simulink model "testRollContSolo"  (R2014a)
settings: Solver=ode3  StartTime=0.0  StopTime=20  FixedStep=0.021  RelTol=1e-3
values from neighbouring files (symbols this model uses):
  armLength = 0.23    [RollDynamics.m]    (also in RollDynamicsPWM-Theta.m; rollDynamics.m)
  enableSaturation = -1    [RollDynamics.m]
  Kforce = Ct*rho*Aprop*2*Whovering*Radius^2    (= 0.344086923283)    [RollDynamics.m]    (also in rollDynamics.m)
  mode = 1    [RollDynamics.m]    (also in RollDynamicsPWM-Theta.m = -1; rollDynamics.m = -1)
  pwmLowerBound = 1001    [RollDynamics.m]    (also in RollDynamicsPWM-Theta.m = 1100; rollDynamics.m = 1000)
  pwmUpperBound = 2000    [RollDynamics.m]    (also in RollDynamicsPWM-Theta.m = 1700; rollDynamics.m = 1800)
  Ts = 0.021    [RollDynamics.m]    (also in RollDynamicsPWM-Theta.m; rollDynamics.m)
  Whovering = 1420    [RollDynamics.m]    (also in RollDynamicsPWM-Theta.m = 750; rollDynamics.m)
undefined symbols (not defined in the file or in its folder): motor_den_tf_discrete, motor_num_tf_discrete, roll_den_tf_discrete, sigbuilder_block
libraries: simulink x2
settings Model: Creator=root  LastModifiedBy=root

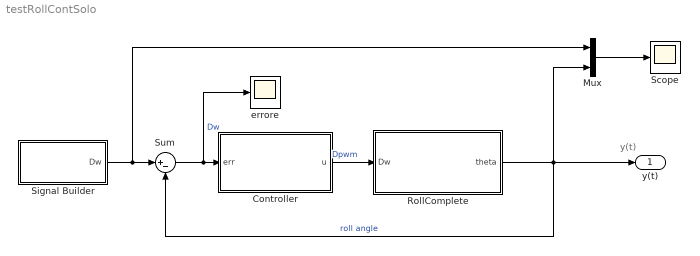
== system testRollContSolo ==
  note: y(t)
  "Controller " : Subsystem
  Mux : Mux  Inputs=2
  "RollComplete " : Subsystem
  Scope : Scope
      settings: TimeRange=10  YMin=-4  YMax=11
  Signal Builder : Subsystem  Tag=STV Subsys  LoadFcn=sigbuilder_block('load');  StartFcn=sigbuilder_block('start');  StopFcn=sigbuilder_block('stop');  ClipboardFcn=sigbuilder_block('clipboard');  mask(Sigbuilder block){}
      mask help: Simulink:masks:SigbuilderBlock_MD
      mask init:
      | if ~strcmp(get_param(bdroot(gcbh),'SimulationStatus'),'stopped') tuvar = sigbuilder_block('maskInit'); end
      settings: CopyFcn=sigbuilder_block('copy');  DeleteFcn=sigbuilder_block('delete');  ModelCloseFcn=sigbuilder_block('modelClose');  PreSaveFcn=sigbuilder_block('preSave');  PauseFcn=sigbuilder_block('pause');  ContinueFcn=sigbuilder_block('continue');  NameChangeFcn=sigbuilder_block('namechange');  OpenFcn=sigbuilder_block('open',[264.8 0 542.4 376 ]);  CloseFcn=sigbuilder_block('close');
      mask Display: plot(0, 0, 100, 100,[2, 2, 32, 32, 2], [68, 8, 8, 68, 68],[32, 2], [38, 38], [32, 19, 2],[53, 60, 44], [32, 17, 17, 2],[16, 16, 31, 31]);txt = getActiveGroup(gcbh);text(2, 100, txt,'verticalAlignment', 'top');
  Sum : Sum  Inputs=|+-
  errore : Scope
      settings: TimeRange=10  YMin=-4  YMax=11
  y(t) : Outport
  wires:
  Signal Builder/1(Dw) -> Mux/1, Sum/1
  Mux/1 -> Scope/1
  "RollComplete "/1("theta ") -> Sum/2, Mux/2, y(t)/1  "roll angle"
  Sum/1 -> errore/1, "Controller "/1("err ")  "Dw"
  "Controller "/1("u ") -> "RollComplete "/1("Dw ")  "Dpwm"

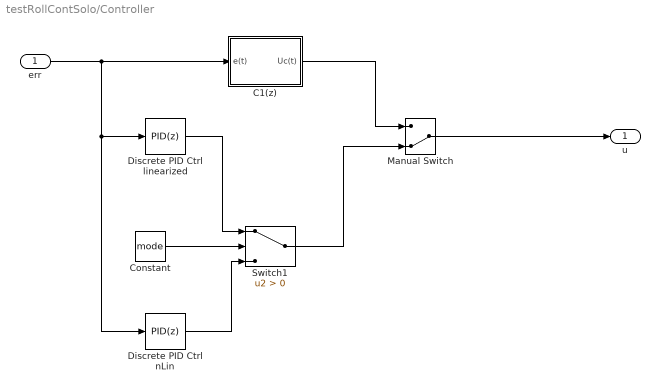
== system testRollContSolo/Controller  ==
  "err " : Inport
  C1(z) : Subsystem
  Constant : Constant  Value=mode
  Discrete PID Ctrl nLin : simulink/Continuous/PID Controller  Controller=PID  TimeDomain=Discrete-time  SampleTime=Ts  IntegratorMethod=Forward Euler  FilterMethod=Forward Euler  Form=Parallel  P=10000  I=0  D=0  N=16.4030945436849  InitialConditionSource=internal  InitialConditionForIntegrator=0  InitialConditionForFilter=0  ExternalReset=none  LimitOutput=off  UpperSaturationLimit=inf  LowerSaturationLimit=-inf  LinearizeAsGain=off  AntiWindupMode=none  Kb=1  TrackingMode=off  Kt=1  PParamMin=[]  PParamMax=[]  IParamMin=[]  IParamMax=[]  DParamMin=[]  DParamMax=[]  NParamMin=[]  NParamMax=[]  KbParamMin=[]  KbParamMax=[]  KtParamMin=[]  KtParamMax=[]  POutMin=[]  POutMax=[]  IOutMin=[]  IOutMax=[]  DOutMin=[]  DOutMax=[]  NOutMin=[]  NOutMax=[]  KbOutMin=[]  KbOutMax=[]  KtOutMin=[]  KtOutMax=[]  IntegratorOutMin=[]  IntegratorOutMax=[]  FilterOutMin=[]  FilterOutMax=[]  SumOutMin=[]  SumOutMax=[]  SumI1OutMin=[]  SumI1OutMax=[]  SumI2OutMin=[]  SumI2OutMax=[]  SumI3OutMin=[]  SumI3OutMax=[]  SumDOutMin=[]  SumDOutMax=[]  SaturationOutMin=[]  SaturationOutMax=[]  IntegratorContinuousStateAttributes=''  IntegratorStateMustResolveToSignalObject=off  IntegratorRTWStateStorageClass=Auto  FilterContinuousStateAttributes=''  FilterStateMustResolveToSignalObject=off  FilterRTWStateStorageClass=Auto
  "Discrete PID Ctrl linearized " : simulink/Continuous/PID Controller  Controller=PID  TimeDomain=Discrete-time  SampleTime=Ts  IntegratorMethod=Forward Euler  FilterMethod=Forward Euler  Form=Parallel  P=54.1819263876867  I=60.1281255168025  D=11.2520369375895  N=27.8352283138862  InitialConditionSource=internal  InitialConditionForIntegrator=0  InitialConditionForFilter=0  ExternalReset=none  LimitOutput=on  UpperSaturationLimit=pwmUpperBound  LowerSaturationLimit=pwmLowerBound  LinearizeAsGain=off  AntiWindupMode=back-calculation  Kb=1  TrackingMode=off  Kt=1  PParamMin=[]  PParamMax=[]  IParamMin=[]  IParamMax=[]  DParamMin=[]  DParamMax=[]  NParamMin=[]  NParamMax=[]  KbParamMin=[]  KbParamMax=[]  KtParamMin=[]  KtParamMax=[]  POutMin=[]  POutMax=[]  IOutMin=[]  IOutMax=[]  DOutMin=[]  DOutMax=[]  NOutMin=[]  NOutMax=[]  KbOutMin=[]  KbOutMax=[]  KtOutMin=[]  KtOutMax=[]  IntegratorOutMin=[]  IntegratorOutMax=[]  FilterOutMin=[]  FilterOutMax=[]  SumOutMin=[]  SumOutMax=[]  SumI1OutMin=[]  SumI1OutMax=[]  SumI2OutMin=[]  SumI2OutMax=[]  SumI3OutMin=[]  SumI3OutMax=[]  SumDOutMin=[]  SumDOutMax=[]  SaturationOutMin=[]  SaturationOutMax=[]  IntegratorContinuousStateAttributes=''  IntegratorStateMustResolveToSignalObject=off  IntegratorRTWStateStorageClass=Auto  FilterContinuousStateAttributes=''  FilterStateMustResolveToSignalObject=off  FilterRTWStateStorageClass=Auto
  Manual Switch : ManualSwitch  CurrentSetting=0
  Switch1 : Switch  Criteria=u2 > Threshold
  "u " : Outport
  wires:
  "err "/1 -> Discrete PID Ctrl nLin/1, "Discrete PID Ctrl linearized "/1, C1(z)/1(e(t))
  Manual Switch/1 -> "u "/1
  Discrete PID Ctrl nLin/1 -> Switch1/3
  C1(z)/1(Uc(t)) -> Manual Switch/1
  "Discrete PID Ctrl linearized "/1 -> Switch1/1
  Constant/1 -> Switch1/2
  Switch1/1 -> Manual Switch/2

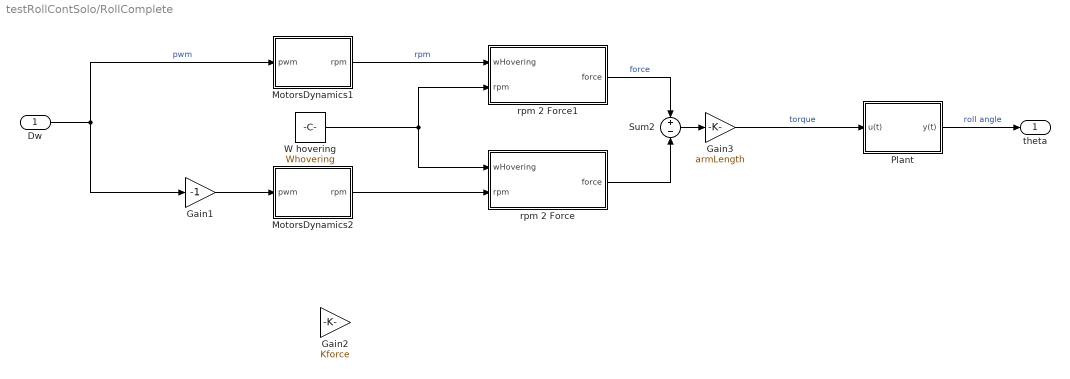
== system testRollContSolo/RollComplete  ==
  "Dw " : Inport
  Gain1 : Gain  Gain=-1  SampleTime=Ts
  Gain2 : Gain  Gain=Kforce  SampleTime=Ts
  Gain3 : Gain  Gain=armLength  SampleTime=Ts
  MotorsDynamics1 : Subsystem
  MotorsDynamics2 : Subsystem
  Plant : Subsystem
  Sum2 : Sum  Inputs=+|-
  W hovering : Constant  Value=Whovering
  rpm 2 Force : Subsystem
  rpm 2 Force1 : Subsystem
  "theta " : Outport
  wires:
  Plant/1(y(t)) -> "theta "/1  "roll angle"
  Sum2/1 -> Gain3/1
  W hovering/1 -> rpm 2 Force1/2(rpm), rpm 2 Force/1(wHovering)
  "Dw "/1 -> MotorsDynamics1/1(pwm), Gain1/1  "pwm"
  Gain1/1 -> MotorsDynamics2/1(pwm)
  MotorsDynamics1/1(rpm) -> rpm 2 Force1/1(wHovering)  "rpm"
  rpm 2 Force1/1(force) -> Sum2/1  "force"
  rpm 2 Force/1(force) -> Sum2/2
  MotorsDynamics2/1(rpm) -> rpm 2 Force/2(rpm)
  Gain3/1 -> Plant/1(u(t))  "torque"

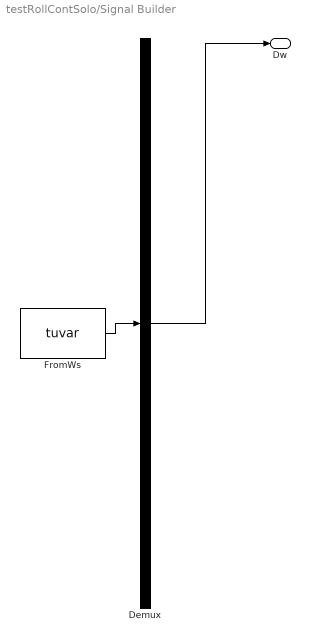
== system testRollContSolo/Signal Builder ==
  Demux : Demux  Tag=STV Demux  Outputs=1
  FromWs : FromWorkspace  Tag=STV FromWs  VariableName=tuvar  SampleTime=0
      SigBuilderData=|
      | common.afterFinalStr = 'Extrapolate'
      | common.sampleTime = 0
      | dataSet.timeRange = [0 10]
      | dataSet.name = 'Group 1'
      | sbobj.Groups.Name = 'Group 1'
      | sbobj.Groups.Signals.Name = 'Dw'
      | sbobj.Groups.Signals.XData = [0 4 4 10]
      | sbobj.Groups.Signals.YData = [0 5.05 10.05 1.95]
  Dw : Outport  Tag=STV Outport
  wires:
  Demux/1 -> Dw/1
  FromWs/1 -> Demux/1

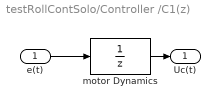
== system testRollContSolo/Controller /C1(z) ==
  e(t) : Inport
  motor Dynamics : DiscreteTransferFcn  Denominator=[1 0 ]  SampleTime=Ts
  Uc(t) : Outport
  wires:
  motor Dynamics/1 -> Uc(t)/1
  e(t)/1 -> motor Dynamics/1

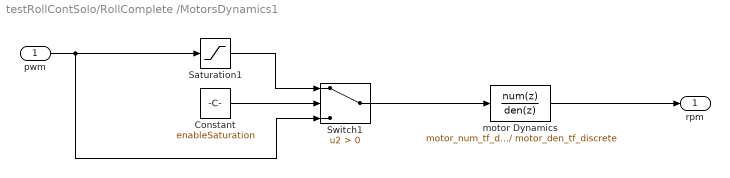
== system testRollContSolo/RollComplete /MotorsDynamics1 ==
  pwm : Inport
  Constant : Constant  Value=enableSaturation
  Saturation1 : Saturate  UpperLimit=pwmUpperBound  LowerLimit=pwmLowerBound  SampleTime=Ts
  Switch1 : Switch  Criteria=u2 > Threshold  SampleTime=Ts
  motor Dynamics : DiscreteTransferFcn  Numerator=motor_num_tf_discrete  Denominator=motor_den_tf_discrete  InitialStates=Whovering  SampleTime=Ts
  rpm : Outport
  wires:
  motor Dynamics/1 -> rpm/1
  Saturation1/1 -> Switch1/1
  Constant/1 -> Switch1/2
  pwm/1 -> Saturation1/1, Switch1/3
  Switch1/1 -> motor Dynamics/1

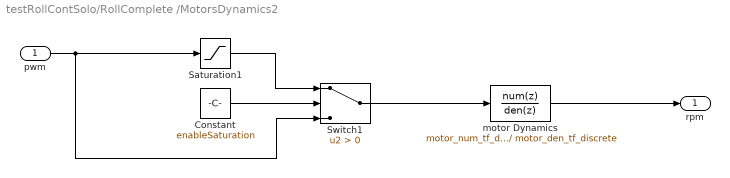
== system testRollContSolo/RollComplete /MotorsDynamics2 ==
  pwm : Inport
  Constant : Constant  Value=enableSaturation
  Saturation1 : Saturate  UpperLimit=pwmUpperBound  LowerLimit=pwmLowerBound  SampleTime=Ts
  Switch1 : Switch  Criteria=u2 > Threshold  SampleTime=Ts
  motor Dynamics : DiscreteTransferFcn  Numerator=motor_num_tf_discrete  Denominator=motor_den_tf_discrete  InitialStates=Whovering  SampleTime=Ts
  rpm : Outport
  wires:
  motor Dynamics/1 -> rpm/1
  Saturation1/1 -> Switch1/1
  Constant/1 -> Switch1/2
  pwm/1 -> Saturation1/1, Switch1/3
  Switch1/1 -> motor Dynamics/1

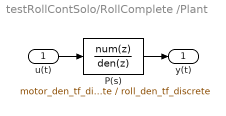
== system testRollContSolo/RollComplete /Plant ==
  u(t) : Inport
  P(s) : DiscreteTransferFcn  Numerator=motor_den_tf_discrete  Denominator=roll_den_tf_discrete  SampleTime=Ts
  y(t) : Outport
  wires:
  P(s)/1 -> y(t)/1
  u(t)/1 -> P(s)/1

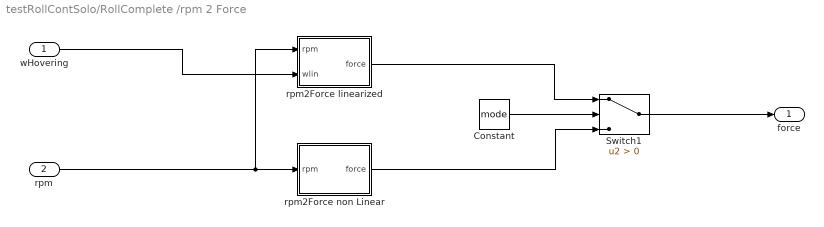
== system testRollContSolo/RollComplete /rpm 2 Force ==
  wHovering : Inport
  rpm : Inport  Port=2
  Constant : Constant  Value=mode
  Switch1 : Switch  Criteria=u2 > Threshold  SampleTime=Ts
  rpm2Force linearized : MATLAB Function  TreatAsAtomicUnit=on
  rpm2Force non Linear : MATLAB Function  TreatAsAtomicUnit=on
  force : Outport
  wires:
  rpm/1 -> rpm2Force linearized/1(rpm), rpm2Force non Linear/1(rpm)
  wHovering/1 -> rpm2Force linearized/2(wlin)
  rpm2Force linearized/1(force) -> Switch1/1
  Constant/1 -> Switch1/2
  rpm2Force non Linear/1(force) -> Switch1/3
  Switch1/1 -> force/1

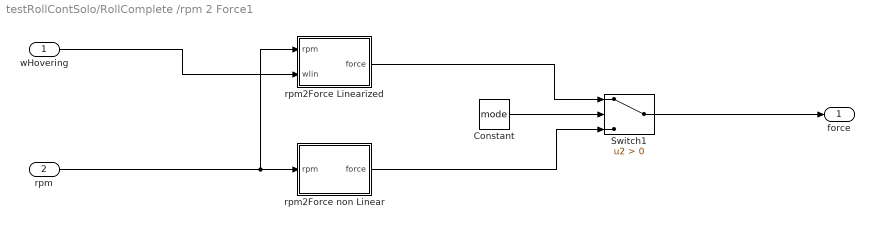
== system testRollContSolo/RollComplete /rpm 2 Force1 ==
  wHovering : Inport
  rpm : Inport  Port=2
  Constant : Constant  Value=mode  SampleTime=Ts
  Switch1 : Switch  Criteria=u2 > Threshold
  rpm2Force Linearized : MATLAB Function  TreatAsAtomicUnit=on
  rpm2Force non Linear : MATLAB Function  TreatAsAtomicUnit=on
  force : Outport
  wires:
  rpm2Force non Linear/1(force) -> Switch1/3
  rpm/1 -> rpm2Force Linearized/1(rpm), rpm2Force non Linear/1(rpm)
  wHovering/1 -> rpm2Force Linearized/2(wlin)
  rpm2Force Linearized/1(force) -> Switch1/1
  Constant/1 -> Switch1/2
  Switch1/1 -> force/1

== matlab function testRollContSolo/RollComplete /rpm 2 Force/rpm2Force non Linear ==
  data: rpm input; force output
function force = fcn(rpm)
%#codegen

% Computing Thrust force. It is the result of vertical forces acting on all
% blade elements of one propeller
Radius = 0.115 % m
Radius_in = 9 % in
Ct = 0.18
rho = 1.225 % kg/m^3
Aprop = pi*Radius^2

% Convert to RPM
Thrust_newton = Ct*rho*Aprop*(rpm)^2*Radius^2;
Thrust_kg = Thrust_newton/9.81


force = Thrust_newton;

== matlab function testRollContSolo/RollComplete /rpm 2 Force1/rpm2Force non Linear ==
  data: rpm input; force output
function force = fcn(rpm)
%#codegen

% Computing Thrust force. It is the result of vertical forces acting on all
% blade elements of one propeller
Radius = 0.115; % m
Radius_in = 9; % in
Ct = 0.18;
rho = 1.225; % kg/m^3
Aprop = pi*Radius^2;

% Convert to RPM
Thrust_newton = Ct*rho*Aprop*(rpm)^2*Radius^2;
Thrust_kg = Thrust_newton/9.81;


force = Thrust_newton;

== matlab function testRollContSolo/RollComplete /rpm 2 Force/rpm2Force linearized ==
  data: rpm input; force output; wlin input
function force = fcn(rpm,wlin)
%#codegen

% Computing Thrust force. It is the result of vertical forces acting on all
% blade elements of one propeller
Radius = 0.115 % m
Radius_in = 9 % in
Ct = 0.18
rho = 1.225 % kg/m^3
Aprop = pi*Radius^2

% Convert to RPM
Thrust_newton = Ct*rho*Aprop*(rpm)*2*wlin*Radius^2;
Thrust_kg = Thrust_newton/9.81


force = Thrust_newton;

== matlab function testRollContSolo/RollComplete /rpm 2 Force1/rpm2Force Linearized ==
  data: rpm input; force output; wlin input
function force = fcn(rpm,wlin)
%#codegen

% Computing Thrust force. It is the result of vertical forces acting on all
% blade elements of one propeller
Radius = 0.115; % m
Radius_in = 9; % in
Ct = 0.18;
rho = 1.225; % kg/m^3
Aprop = pi*Radius^2;

% Convert to RPM
Thrust_newton = Ct*rho*Aprop*(rpm)*2*wlin*Radius^2;
Thrust_kg = Thrust_newton/9.81;


force = Thrust_newton;
